simulink model "rtwdemo_lct_fixpt_signals"  (Simulink 7.6)
settings: Solver=FixedStepDiscrete  StartTime=0.0  StopTime=10.0  FixedStep=0.1  RelTol=1e-3
PreLoadFcn:
  | load rtwdemo_lct_data.mat
undefined symbols (not defined in the file or in its folder): myFixpt
libraries: rtwdemowidgets x1
Description:
  | Fixed Point Signals
settings Model: MinMaxOverflowLogging=MinMaxAndOverflow  Creator=The MathWorks Inc.  ExtModeAutoUpdateStatusClock=off
settings MATStruct: SampleTime=0.1  Offset=0  Priority=[20.0]
settings DataIOCC: SaveOutput=off  SaveTime=off  SignalLoggingName=logsOut
settings OptimizationCC: InlineParams=on  InlineInvariantSignals=on  PassReuseOutputArgsAs=Individual arguments  StateBitsets=on  DataBitsets=on  UseTempVars=on  ZeroExternalMemoryAtStartup=off  ZeroInternalMemoryAtStartup=off  NoFixptDivByZeroProtection=on  EfficientFloat2IntCast=on  EfficientMapNaN2IntZero=off  OptimizeModelRefInitCode=on  LifeSpan=1
settings DebuggingCC: SolverPrmCheckMsg=none  StrictBusMsg=ErrorOnBusTreatedAsVector
settings HardwareCC: ProdBitPerLong=64  ProdEndianess=LittleEndian  ProdWordSize=64  ProdHWDeviceType=Specified  TargetIntDivRoundTo=Zero  TargetEndianess=LittleEndian  TargetHWDeviceType=Generic->MATLAB Host Computer
settings RTWCC: SystemTargetFile=ert.tlc  TemplateMakefile=ert_default_tmf  Description=Real-Time Workshop Embedded Coder (no auto configuration)  GenerateReport=on  RTWVerbose=off  ProcessScript=ert_make_rtw_hook  IncludeHyperlinkInReport=on  LaunchReport=on  GenerateTraceInfo=on  GenerateTraceReport=on  GenerateTraceReportSl=on  GenerateTraceReportSf=on  GenerateTraceReportEml=on
settings CodeAppCC: ForceParamTrailComments=on  IgnoreCustomStorageClasses=off  IgnoreTestpoints=on  SimulinkDataObjDesc=on  CustomSymbolStrGlobalVar=rt$N$M  CustomSymbolStrType=$N$M  CustomSymbolStrFcn=$N$M$F  CustomSymbolStrMacro=$N$M  InsertBlockDesc=on
settings ERTTargetCC: MultiwordLength=2048  GenerateSampleERTMain=on  IncludeMdlTerminateFcn=off  SupportNonFinite=off  SupportComplex=off  InlinedParameterPlacement=NonHierarchical  ERTCustomFileTemplate=example_file_process.tlc  ConvertIfToSwitch=off

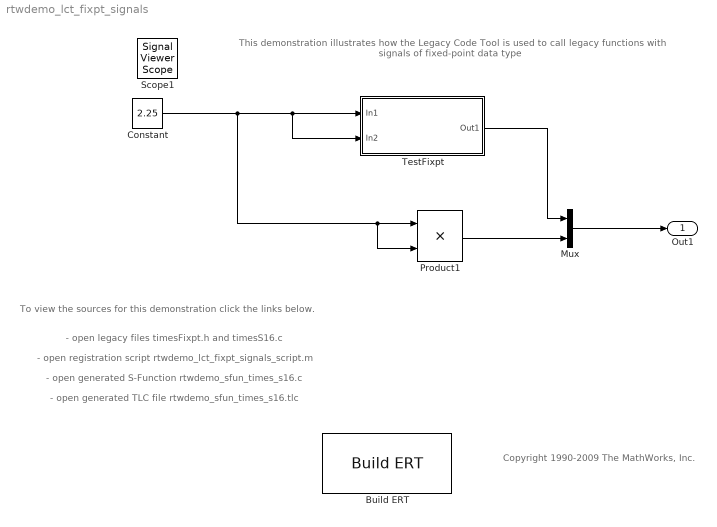
== system rtwdemo_lct_fixpt_signals ==
  note: Copyright 1990-2009 The MathWorks, Inc.
  note: This demonstration illustrates how the Legacy Code Tool is used to
      | call legacy functions with signals of fixed-point data type
  note: - open legacy files timesFixpt.h and timesS16.c
  note: To view the sources for this demonstration
      | click the links below.
  note: - open registration script rtwdemo_lct_fixpt_signals_script.m
  note: - open generated S-Function rtwdemo_sfun_times_s16.c
  note: - open generated TLC file rtwdemo_sfun_times_s16.tlc
  Build ERT : rtwdemowidgets/Build ERT  SystemSampleTime=-1  attrib_overrides={}
  Constant : Constant  Value=2.25  OutDataTypeStr=myFixpt  SampleTime=0.1
  Mux : Mux  Inputs=2
  Product1 : Product  OutDataTypeStr=myFixpt
  TestFixpt : Subsystem
  Out1 : Outport
  Scope1 : SignalViewerScope  IOType=viewer  RefreshTime=0.035000
      settings: YMin=4  YMax=6
  wires:
  Constant/1 -> Product1/1, Product1/2, TestFixpt/1(In1), TestFixpt/2(In2)
  Mux/1 -> Out1/1
  Product1/1 -> Mux/2
  TestFixpt/1(Out1) -> Mux/1

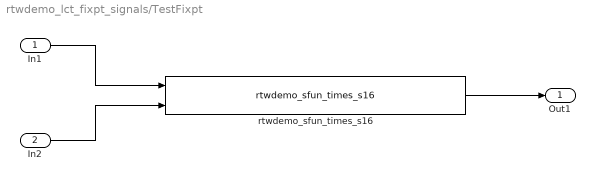
== system rtwdemo_lct_fixpt_signals/TestFixpt ==
  In1 : Inport  OutDataTypeStr=myFixpt
  In2 : Inport  Port=2  OutDataTypeStr=myFixpt
  rtwdemo_sfun_times_s16 : S-Function  FunctionName=rtwdemo_sfun_times_s16  Parameters=SParameter1  EnableBusSupport=off  mask(Legacy Function){SFunctionSpec=myFixpt y1 = timesS16(myFixpt u1, myFixpt u2, uint8 p1), SParameter1=uint8(myFixpt.FractionLength), ShowSpec=on}
      mask prompts: SParameter1 "P1:"; ShowSpec "Display function specification"
      mask help:
      | This block allows you to call the legacy functions specified by the following Legacy Code Tool definition:
      | def.SFunctionName = 'rtwdemo_sfun_times_s16';
      | def.OutputFcnSpec = 'myFixpt y1 = timesS16(myFixpt u1, myFixpt u2, uint8 p1)';
      | def.HeaderFiles = {'timesFixpt.h'};
      | def.SourceFiles = {'timesS16.c'};
      | def.IncPaths = {'sldemo_lct_src'};
      | def.SrcPaths = {'sldemo_lct_src'};
      mask Help: <p>This block was generated automatically by the Legacy Code Tool. For detailed help on this tool, call<a href="matlab:legacy_code('help')"> legacy_code('help')</a>.</p>
      mask CallbackString:
      | ||if strcmp(get_param(gcbh, 'ShowSpec'), 'on')
      |   set_param(gcbh, 'MaskDisplay', sprintf('fprintf(''%s'');', get_param(gcbh, 'SFunctionSpec')));
      | else
      |   set_param(gcbh, 'MaskDisplay', sprintf('fprintf(''%s'');', get_param(gcbh, 'FunctionName')));
      | end
      mask Display: fprintf('myFixpt y1 = timesS16(myFixpt u1, myFixpt u2, uint8 p1)');
  Out1 : Outport
  wires:
  rtwdemo_sfun_times_s16/1 -> Out1/1
  In1/1 -> rtwdemo_sfun_times_s16/1
  In2/1 -> rtwdemo_sfun_times_s16/2
